simulink model "torques_example"  (R2024b)
settings: Solver=FixedStepAuto  StartTime=0.0  StopTime=inf  FixedStep=0.0005  RelTol=1e-3
libraries: BeamNG_interface x1
settings Model: Creator=matti  LastModifiedBy=pschr
settings OptimizationCC: ReuseModelBlockBuffer=off
settings DebuggingCC: ArithmeticOperatorsInVariantConditions=warning
settings SFSimCC: CustomCodeUndefinedFunction=UseInterfaceOnly
settings RTWCC: GPUComputeCapability=3.5

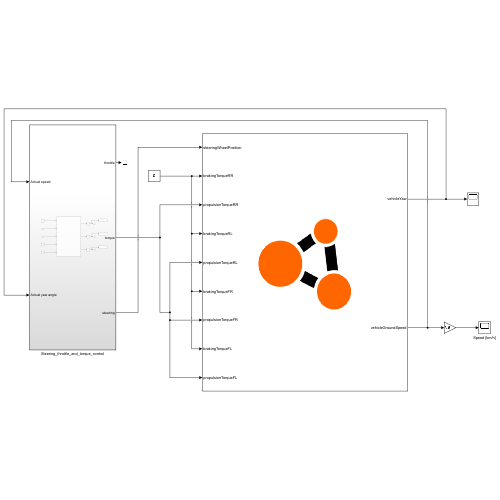
[thumbnail: Simulink's stored preview of the top-level diagram]
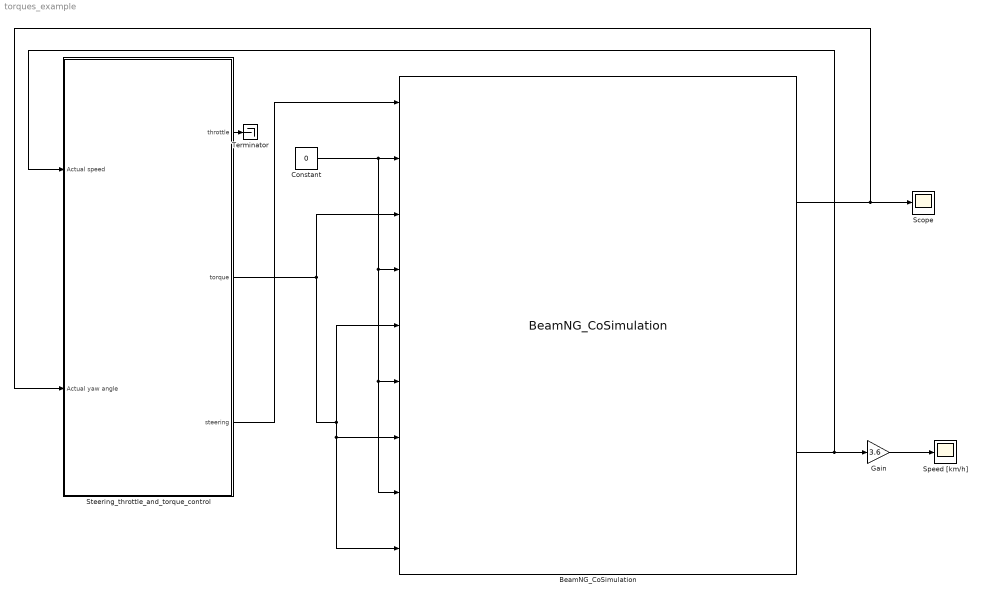
== system torques_example ==
  BeamNG_CoSimulation : BeamNG_interface/BeamNG_CoSimulation  csvFilePath='torques_example.csv'
      settings: SourceProductName=BeamNG
  Constant : Constant  Value=0
  Gain : Gain  Gain=3.6
  Scope : Scope
  Speed [km/h] : Scope
  Steering_throttle_and_torque_control : Subsystem
  Terminator : Terminator
  wires:
  BeamNG_CoSimulation/2 -> Steering_throttle_and_torque_control/1(Actual speed), Gain/1
  BeamNG_CoSimulation/1 -> Steering_throttle_and_torque_control/2(Actual yaw angle), Scope/1
  Steering_throttle_and_torque_control/2(torque) -> BeamNG_CoSimulation/9, BeamNG_CoSimulation/7, BeamNG_CoSimulation/5, BeamNG_CoSimulation/3
  Constant/1 -> BeamNG_CoSimulation/6, BeamNG_CoSimulation/8, BeamNG_CoSimulation/4, BeamNG_CoSimulation/2
  Steering_throttle_and_torque_control/1(throttle) -> Terminator/1
  Gain/1 -> Speed [km/h]/1
  Steering_throttle_and_torque_control/3(steering) -> BeamNG_CoSimulation/1

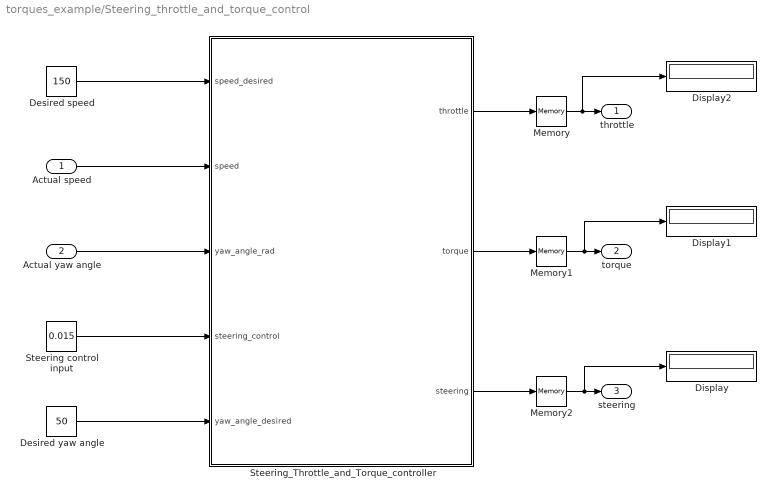
== system torques_example/Steering_throttle_and_torque_control ==
  Actual speed : Inport
  Actual yaw angle : Inport  Port=2
  Desired speed : Constant  Value=150
  Desired yaw angle : Constant  Value=50
  Display : Display
  Display1 : Display
  Display2 : Display
  Memory : Memory
  Memory1 : Memory
  Memory2 : Memory
  Steering control input : Constant  Value=0.015
  Steering_Throttle_and_Torque_controller : MATLAB Function  TreatAsAtomicUnit=on
  throttle : Outport
  torque : Outport  Port=2
  steering : Outport  Port=3
  wires:
  Memory2/1 -> Display/1, steering/1
  Steering_Throttle_and_Torque_controller/2(torque) -> Memory1/1
  Memory1/1 -> Display1/1, torque/1
  Memory/1 -> throttle/1, Display2/1
  Steering_Throttle_and_Torque_controller/3(steering) -> Memory2/1
  Steering control input/1 -> Steering_Throttle_and_Torque_controller/4(steering_control)
  Actual speed/1 -> Steering_Throttle_and_Torque_controller/2(speed)
  Actual yaw angle/1 -> Steering_Throttle_and_Torque_controller/3(yaw_angle_rad)
  Steering_Throttle_and_Torque_controller/1(throttle) -> Memory/1
  Desired yaw angle/1 -> Steering_Throttle_and_Torque_controller/5(yaw_angle_desired)
  Desired speed/1 -> Steering_Throttle_and_Torque_controller/1(speed_desired)

== matlab function torques_example/Steering_throttle_and_torque_control/Steering_Throttle_and_Torque_controller ==
  data: throttle output; torque output; steering output; speed_desired input; speed input; yaw_angle_rad input; steering_control input; yaw_angle_desired input
function [throttle,torque,steering] = Controller(speed_desired,speed,yaw_angle_rad,steering_control,yaw_angle_desired)
% wrapper for controller in m-file
[throttle,torque,steering] = controller(speed_desired,speed,yaw_angle_rad,steering_control,yaw_angle_desired);
end
